simulink model "Compliance_Jawwad"  (R2023a)
settings: Solver=VariableStepAuto  StartTime=0.0  StopTime=3  RelTol=1e-3
values from neighbouring files (symbols this model uses):
  Kd = diag([70,70,70,10,10,10])    [parameters.m]
  Kp = diag([250,250,250,30,30,30])    [parameters.m]
  xd = [H(1:3,4); eulers']    [parameters.m]
undefined symbols (not defined in the file or in its folder): parms
settings Model: Creator=uzair  LastModifiedBy=syedj
settings OptimizationCC: ReuseModelBlockBuffer=off

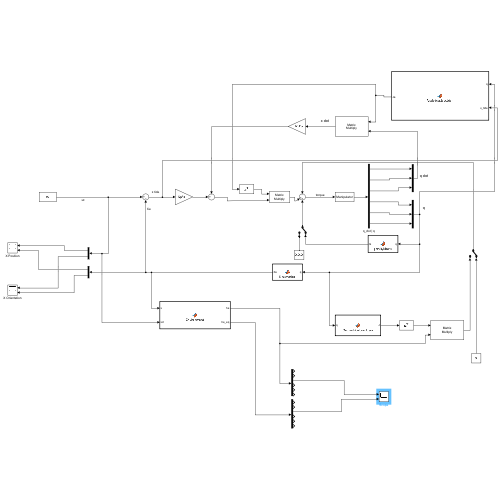
[thumbnail: Simulink's stored preview of the top-level diagram]
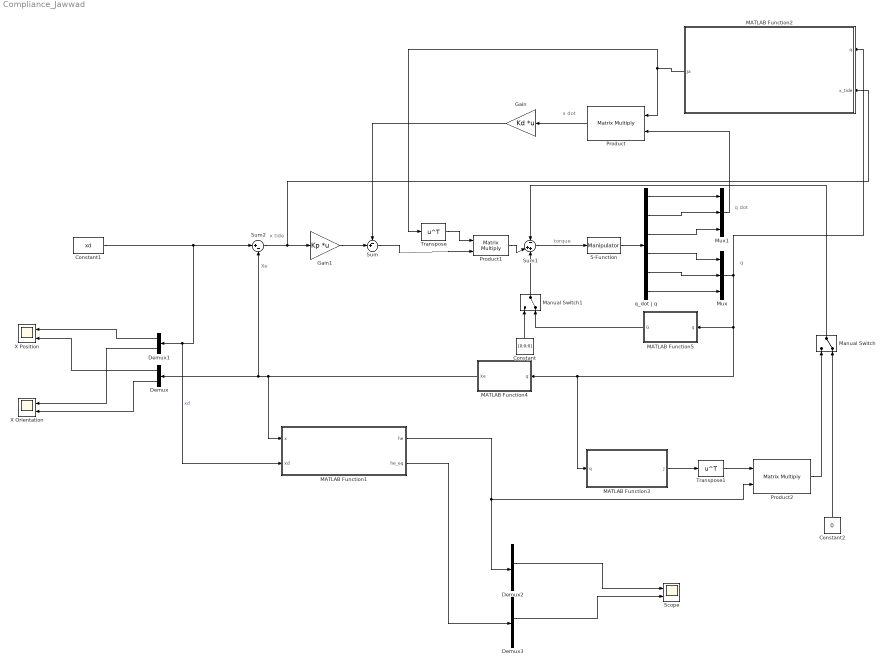
== system Compliance_Jawwad ==
  note: torque
  note: x tide
  note: q
  note: q dot
  note: Xe
  note: x dot
  Constant : Constant  Value=[0;0;0]
  Constant1 : Constant  Value=xd  VectorParams1D=off
  Constant2 : Constant  Value=0
  Demux : Demux  Outputs=2
  Demux1 : Demux  Outputs=2
  Demux2 : Demux  Outputs=6
  Demux3 : Demux  Outputs=6
  Gain : Gain  Gain=Kd  Multiplication=Matrix(K*u)
  Gain1 : Gain  Gain=Kp  Multiplication=Matrix(K*u)
  MATLAB Function1 : MATLAB Function  TreatAsAtomicUnit=on
  MATLAB Function2 : MATLAB Function  TreatAsAtomicUnit=on
  MATLAB Function3 : MATLAB Function  TreatAsAtomicUnit=on
  MATLAB Function4 : MATLAB Function  TreatAsAtomicUnit=on
  MATLAB Function5 : MATLAB Function  TreatAsAtomicUnit=on
  Manual Switch : ManualSwitch  CurrentSetting=0
  Manual Switch1 : ManualSwitch  CurrentSetting=0
  Mux : Mux  Inputs=3
  Mux1 : Mux  Inputs=3
  Product : Product  Multiplication=Matrix(*)
  Product1 : Product  Multiplication=Matrix(*)
  Product2 : Product  Multiplication=Matrix(*)
  S-Function : S-Function  FunctionName=Manipulator  Parameters=params  SFunctionDeploymentMode=off  EnableBusSupport=off
  Scope : Scope  NumInputPorts=2
  Sum : Sum  Inputs=-+|
  Sum1 : Sum  Inputs=-|++
  Sum2 : Sum  Inputs=|+-
  Transpose : Math  Operator=transpose  SignedPower=on  RndMeth=Zero
  Transpose1 : Math  Operator=transpose  SignedPower=on  RndMeth=Zero
  X Orientation : Scope  NumInputPorts=2
  X Position : Scope  NumInputPorts=2
  q_dot | q : Demux  Outputs=6
  wires:
  S-Function/1 -> q_dot | q/1
  q_dot | q/6 -> Mux/3
  q_dot | q/5 -> Mux/2
  q_dot | q/4 -> Mux/1
  q_dot | q/1 -> Mux1/1
  q_dot | q/2 -> Mux1/2
  q_dot | q/3 -> Mux1/3
  Gain/1 -> Sum/1
  Sum1/1 -> S-Function/1
  Mux/1 -> MATLAB Function2/1(q), MATLAB Function5/1(q), MATLAB Function3/1(q), MATLAB Function4/1(q)
  Gain1/1 -> Sum/2
  Sum2/1 -> MATLAB Function2/2(x_tide), Gain1/1
  MATLAB Function5/1(G) -> Manual Switch1/2
  Constant/1 -> Manual Switch1/1
  Mux1/1 -> Product/2
  MATLAB Function2/1(Ja) -> Transpose/1, Product/1
  MATLAB Function4/1(Xe) -> Demux/1, Sum2/2, MATLAB Function1/1(x)
  Constant1/1 -> MATLAB Function1/2(xd), Demux1/1, Sum2/1  "xd"
  Demux1/1 -> X Position/1
  Demux/1 -> X Position/2
  Product1/1 -> Sum1/2
  Sum/1 -> Product1/2
  Demux1/2 -> X Orientation/1
  Demux/2 -> X Orientation/2
  Product/1 -> Gain/1
  Transpose/1 -> Product1/1
  MATLAB Function3/1(J) -> Transpose1/1
  Transpose1/1 -> Product2/1
  MATLAB Function1/1(he) -> Demux2/1, Product2/2
  Demux2/3 -> Scope/1
  MATLAB Function1/2(he_eq) -> Demux3/1
  Demux3/3 -> Scope/2
  Manual Switch/1 -> Sum1/1
  Product2/1 -> Manual Switch/1
  Constant2/1 -> Manual Switch/2
  Manual Switch1/1 -> Sum1/3

== matlab function Compliance_Jawwad/MATLAB Function1 ==
  data: x input; he output; xd input; parms parameter; Kp parameter; he_eq output
function [he,he_eq]= Environment(x, xd, parms, Kp)
    if(x(parms.plane_axis) >= parms.plane_pos(parms.plane_axis))
        xr = parms.plane_pos;

        xdes = zeros(6,1);
        xdes(parms.plane_axis) = xd(parms.plane_axis);

        xe = zeros(6,1);
        xe(parms.plane_axis) = x(parms.plane_axis);

        he = parms.Ke * (xe - xr);

        he_eq = pinv(eye(6) + parms.Ke*pinv(Kp))*parms.Ke*(xdes - xr);

    else
        he = zeros(6,1);
        he_eq = zeros(6,1);
    end
end

== matlab function Compliance_Jawwad/MATLAB Function5 ==
  data: q input; G output; params parameter
function G = gravityMatrix(q, params)
    q1 = q(1);
    q2 = q(2);
    q3 = q(3);
    
    g = params.g;

    m1 = params.m(1);
    m2 = params.m(2);
    m3 = params.m(3);

    a1 = 0.02;
    a2 = 0.03;
    a3 = 0.01;
    b1 = 0.1256;
    b2 = 0.03;
    b3 = 0.01;
    c1 = 0.4;
    c2 = 0.46;
    c3 = 0.15;

    G = [(c1*g*m1*cos(q1))/2 + g*m2*cos(q1)*(c1 - c2/2) + g*m3*cos(q1)*(c1 + c3/2 + q3)
        0;
        g*m3*sin(q1)];
end

== matlab function Compliance_Jawwad/MATLAB Function2 ==
  data: q input; Ja output; x_tide input
function Ja = AnalyticalJacobian(q,x_tide)

    %use desired frame reference, 1 is desired frame
    flag = 0;

    q1 = q(1);
    q2 = q(2);
    q3 = q(3);

    r1 = 0.4;
    a1 = 0.02;
    a2 = 0.03;
    a3 = 0.01;
    b1 = 0.1256;
    b2 = 0.03;
    b3 = 0.01;
    c1 = 0.4;
    c2 = 0.46;
    c3 = 0.15;

    if flag == 0
     H = [[0, -sin(q1), cos(q1),              cos(q1)*(c1 + c3 + q3)]
[1,        0,       0,                           - c2 - q2]
[0,  cos(q1), sin(q1), r1 + sin(q1)*(c3 + q3) + c1*sin(q1)]
[0,        0,       0,                                   1]];

        eulers = rotm2eul(H(1:3,1:3), "ZYZ");


        phi1 = eulers(1);
        phi2 = eulers(2);
        phi3 = eulers(3); %not used

      Ja_m = [
[        -sin(q1)*(c1 + c3 + q3),  0, cos(q1)]
[                              0, -1,       0]
[         cos(q1)*(c1 + c3 + q3),  0, sin(q1)]
[(cos(phi2)*sin(phi1))/sin(phi2),  0,       0]
[                     -cos(phi1),  0,       0]
[           -sin(phi1)/sin(phi2),  0,       0]
];


        Ja = Ja_m;

    else

    J = [
    [-sin(q1)*(c1 + c3 + q3),  0, cos(q1)]
    [                      0, -1,       0]
    [ cos(q1)*(c1 + c3 + q3),  0, sin(q1)]
    [                      0,  0,       0]
    [                     -1,  0,       0]
    [                      0,  0,       0]
    ];

    euler = x_tide(4:6);

        phi1 = euler(1);
        phi2 = euler(2);

        T = [[0, -sin(phi1) ,    cos(phi1)*sin(phi2)];
                 [0,  cos(phi1) ,   sin(phi1)*sin(phi2)];
                 [1,               0  ,    cos(phi2)]];

        Rd = eul2rotm(x_tide(4:6)',"ZYZ");

        Ta = [[eye(3), zeros(3)];
              [zeros(3), T]];

        Ja = -pinv(Ta)*[[Rd', zeros(3)]; 
                        [zeros(3), Rd']] * J;

    end
end

== matlab function Compliance_Jawwad/MATLAB Function3 ==
  data: q input; J output
function J = GeomatricalJacobian(q)
q1 = q(1);
q2 = q(2);
q3 = q(3);
c1 = 0.4;
c2 = 0.3;
c3 = 0.16;
r1 = 0.15;

    J = [
[-sin(q1)*(c1 + c3 + q3),  0, cos(q1)]
[                      0, -1,       0]
[ cos(q1)*(c1 + c3 + q3),  0, sin(q1)]
[                      0,  0,       0]
[                     -1,  0,       0]
[                      0,  0,       0]
];
    
end

== matlab function Compliance_Jawwad/MATLAB Function4 ==
  data: q input; Xe output
function Xe = Kinematics(q)
    q1 = q(1);
    q2 = q(2);
    q3 = q(3);
    
    r1 = 0.4;
    a1 = 0.02;
    a2 = 0.03;
    a3 = 0.01;
    b1 = 0.1256;
    b2 = 0.03;
    b3 = 0.01;
    c1 = 0.4;
    c2 = 0.46;
    c3 = 0.15;


 H = [[0, -sin(q1), cos(q1),              cos(q1)*(c1 + c3 + q3)]
[1,        0,       0,                           - c2 - q2]
[0,  cos(q1), sin(q1), r1 + sin(q1)*(c3 + q3) + c1*sin(q1)]
[0,        0,       0,                                   1]];


    eulers = rotm2eul(H(1:3,1:3), "ZYZ");

    Xe = [H(1:3,4); eulers'];
end
